simulink model "gm_sampleModel1758_5_sub"  (R2023a)
settings: Solver=VariableStepAuto  StartTime=0.0  StopTime=10.0  RelTol=1e-3
libraries: simulink x1
settings Model: Creator=user1  LastModifiedBy=user1
settings OptimizationCC: BlockReduction=off  ConditionallyExecuteInputs=off
settings DebuggingCC: InheritedTsInSrcMsg=none

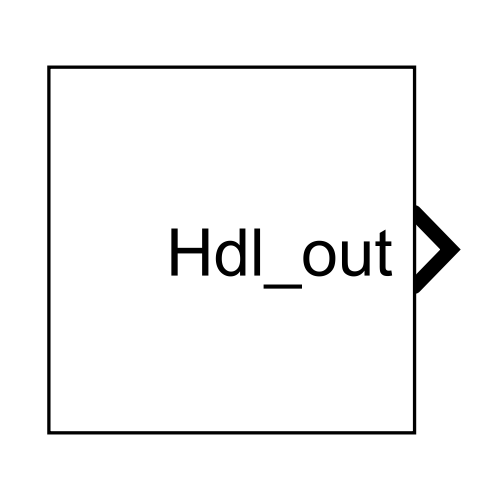
[thumbnail: Simulink's stored preview of the top-level diagram]
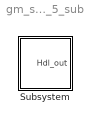
== system gm_sampleModel1758_5_sub ==
  Subsystem : Subsystem

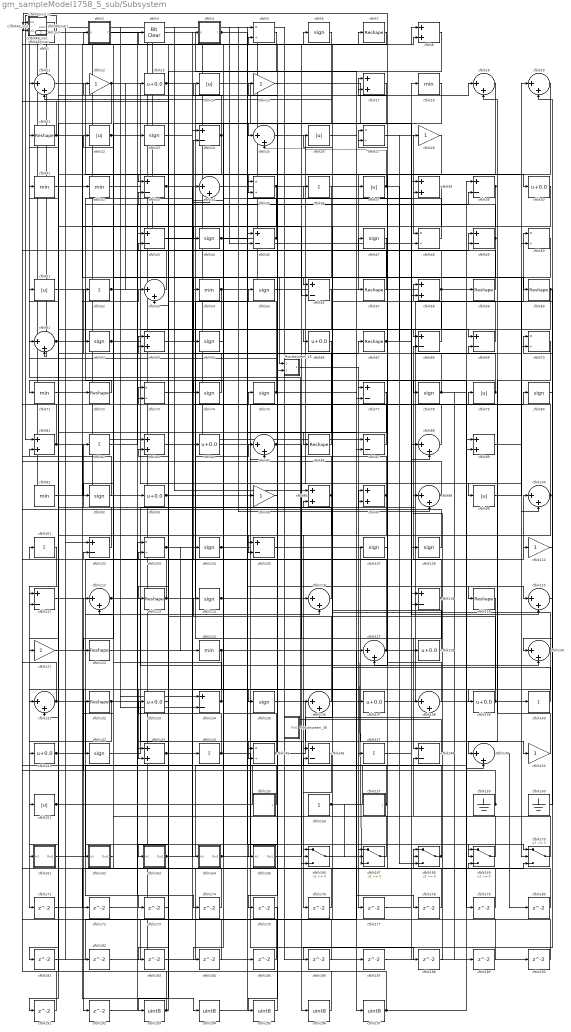
== system gm_sampleModel1758_5_sub/Subsystem ==
  Mysubsystem_38 : Subsystem
  Mysubsystem_45 : Subsystem
  cfblk1 : Logic  AllPortsSameDT=off  OutDataTypeStr=boolean
  cfblk{11,19..20,25,34,53,61,85,88,98,100,112,116,120,127,130..131,136,138,149} (20 alike) : Sum  Inputs=|++  OutDataTypeStr=uint8
  cfblk{36,52,82,101,140,144,147} (7 alike) : Sum  Inputs=+  OutDataTypeStr=uint8
  cfblk{24,33,39,43,45,49,56,68..69,77,87,102,105,111,118,134,146,148} (18 alike) : Sum  Inputs=+-  OutDataTypeStr=uint8
  cfblk{5,27,35,48,50,70,73,103,145} (9 alike) : Product  Inputs=*/  OutDataTypeStr=uint8  RndMeth=Zero  SaturateOnIntegerOverflow=on
  cfblk{6,23,44,47,55,62,64,74..75,78,80,92,104,107..108,114,135,142} (18 alike) : Signum
  cfblk106_inst : Subsystem
  cfblk109_inst : Subsystem
  cfblk10_inst : Subsystem
  cfblk{12,15,28,95,110,121,150} (7 alike) : Gain  OutDataTypeStr=uint8
  cfblk{7,21,57,59..60,67,72,86,113,119,122,132} (12 alike) : Reshape
  cfblk115_inst : Subsystem
  cfblk117_inst : Subsystem
  cfblk{18,31..32,54,71,91,124} (7 alike) : MinMax  OutDataTypeStr=uint8
  cfblk125_inst : Subsystem
  cfblk{13,40,66,84,93,128,133,137,139,141} (10 alike) : Bias  Bias=0.0  SaturateOnIntegerOverflow=off
  cfblk129_inst : Subsystem
  cfblk{14,22,26,37,51,79,99,151} (8 alike) : Abs  OutDataTypeStr=uint8  SaturateOnIntegerOverflow=off
  cfblk{8,17,38,58,63,81,83,89,96..97,143} (11 alike) : Sum  OutDataTypeStr=uint8
  cfblk155 : Subsystem  mask(Counter Limited){uplimit=double(7), tsamp=double(-1)}
      mask prompts: uplimit "Simulink:masks:UpperLimit_MP"; tsamp "Simulink:masks:SampleTime_MP"
      mask help: Simulink:masks:CounterLimited_MD
      mask init:
      | nbits = double(8);
      | tsamp = double(-1);
      | uplimit = double(7);
  cfblk156 : Constant  OutDataTypeStr=uint8  SampleTime=-1
  cfblk157 : Subsystem  mask(Counter Free-Running){NumBits=double(16), tsamp=double(-1)}
      mask prompts: NumBits "Simulink:masks:NumberOfBits_MP"; tsamp "Simulink:masks:SampleTime_MP"
      mask help: Simulink:masks:CounterFreeRunning_MD
  cfblk159 : Ground
  cfblk160 : Ground
  cfblk161 : Subsystem
  cfblk162 : Subsystem
  cfblk163 : Subsystem
  cfblk164 : Subsystem
  cfblk165 : Subsystem
  cfblk{166..170} (5 alike) : Switch  OutDataTypeStr=uint8  SaturateOnIntegerOverflow=off  InputSameDT=off
  cfblk16_inst : Subsystem
  cfblk{171..192} (22 alike) : Delay  SampleTime=1
  cfblk{193..197} (5 alike) : DataTypeConversion  OutDataTypeStr=uint8  SaturateOnIntegerOverflow=off  RndMeth=Floor
  cfblk2 : Subsystem  mask(Detect Fall Nonpositive){vinit=double(0), InputProcessing=Elements as channels (sample based), OutDataTypeStr=uint8}
      mask prompts: vinit "Simulink:masks:InitialCondition_MP"; InputProcessing "Simulink:masks:InputProcessing_MP"; OutDataTypeStr "Simulink:masks:OutputDataType_MP"
      mask help: Simulink:masks:DetectFallNonpositive_MD
      mask init:
      | InputProcessing = 'Elements as channels (sample based)';
      | OutDataTypeStr = 'uint8';
      | vinit = double(0);
      mask TypeOptions InputProcessing: Simulink:masks:ColumnsAsChannelsFrameBased | Simulink:masks:ElementsAsChannelsSampleBased
      mask TypeOptions OutDataTypeStr: Simulink:masks:uint8 | Simulink:masks:boolean
      mask Display: fprintf('U <= 0\n&  NOT\nU/z <= 0')
  cfblk29_inst : Subsystem
  cfblk3 : simulink/Logic and Bit Operations/Bit Clear  iBit=0
      settings: LibrarySourceBlock=|
      | hdlsllib/Logic and Bit
      | Operations/Bit Clear
  cfblk30_inst : Subsystem
  cfblk4 : Subsystem  mask(Detect Rise Nonnegative){vinit=double(0), InputProcessing=Elements as channels (sample based), OutDataTypeStr=uint8}
      mask prompts: vinit "Simulink:masks:InitialCondition_MP"; InputProcessing "Simulink:masks:InputProcessing_MP"; OutDataTypeStr "Simulink:masks:OutputDataType_MP"
      mask help: Simulink:masks:DetectRiseNonnegative_MD
      mask init:
      | InputProcessing = 'Elements as channels (sample based)';
      | OutDataTypeStr = 'uint8';
      | vinit = double(0);
      mask TypeOptions InputProcessing: Simulink:masks:ColumnsAsChannelsFrameBased | Simulink:masks:ElementsAsChannelsSampleBased
      mask TypeOptions OutDataTypeStr: Simulink:masks:uint8 | Simulink:masks:boolean
      mask Display: fprintf('U >= 0\n&  NOT\nU/z >= 0')
  cfblk41_inst : Subsystem
  cfblk42_inst : Subsystem
  cfblk46_inst : Subsystem
  cfblk90_inst : Subsystem
  cfblk94_inst : Subsystem
  cfblk9_inst : Subsystem
  Hdl_out : Outport  OutDataTypeStr=uint8  SampleTime=1
  wires:
  Mysubsystem_38/1(Out1) -> cfblk1/2
  Mysubsystem_45/1(Out1) -> cfblk177/1
  cfblk1/1 -> cfblk81/1
  cfblk10_inst/1(out1) -> cfblk134/1
  cfblk100/1 -> cfblk46_inst/2(in2), cfblk176/1
  cfblk101/1 -> cfblk171/1
  cfblk102/1 -> cfblk82/1
  cfblk103/1 -> cfblk97/1, cfblk55/1, cfblk124/1
  cfblk104/1 -> cfblk85/2, cfblk80/1
  cfblk105/1 -> cfblk150/1
  cfblk106_inst/1(out1) -> cfblk93/1, cfblk102/1
  cfblk107/1 -> cfblk27/1
  cfblk108/1 -> cfblk129_inst/1(in1)
  cfblk109_inst/1(out1) -> cfblk61/2, cfblk117_inst/1(in1), cfblk91/1
  cfblk11/1 -> cfblk40/1
  cfblk110/1 -> cfblk58/1
  cfblk111/1 -> cfblk100/1
  cfblk112/1 -> cfblk130/2, cfblk50/1
  cfblk113/1 -> cfblk85/1, cfblk117_inst/2(in2)
  cfblk114/1 -> cfblk116/1, cfblk110/1
  cfblk115_inst/1(out1) -> cfblk42_inst/2(in2), cfblk185/1
  cfblk116/1 -> cfblk31/1
  cfblk117_inst/1(out1) -> cfblk140/1, cfblk32/1
  cfblk118/1 -> cfblk68/2, cfblk148/1
  cfblk119/1 -> cfblk139/1
  cfblk12/1 -> cfblk149/2, cfblk121/1
  cfblk120/1 -> cfblk186/1
  cfblk121/1 -> cfblk116/2
  cfblk122/1 -> cfblk144/1
  cfblk124/1 -> cfblk167/3, cfblk143/2, cfblk192/1
  cfblk125_inst/1(out1) -> cfblk72/1, cfblk59/1
  cfblk127/1 -> cfblk69/2, cfblk22/1, cfblk73/1
  cfblk128/1 -> cfblk46_inst/1(in1)
  cfblk129_inst/1(out1) -> cfblk87/1, cfblk23/1
  cfblk13/1 -> cfblk25/1, cfblk35/2, cfblk187/1
  cfblk130/1 -> cfblk11/2, cfblk172/1
  cfblk131/1 -> cfblk42_inst/1(in1), cfblk173/1
  cfblk132/1 -> cfblk196/1, cfblk151/1, cfblk181/1
  cfblk133/1 -> cfblk163/1(In1)
  cfblk134/1 -> cfblk83/2, cfblk2/1(U)
  cfblk135/1 -> cfblk147/1
  cfblk136/1 -> cfblk63/1
  cfblk137/1 -> cfblk20/1
  cfblk138/1 -> cfblk115_inst/1(in1)
  cfblk139/1 -> cfblk131/1, cfblk114/1
  cfblk14/1 -> cfblk88/2
  cfblk140/1 -> cfblk6/1
  cfblk141/1 -> cfblk45/2, cfblk24/2, cfblk166/2
  cfblk142/1 -> cfblk79/1
  cfblk143/1 -> cfblk75/1, cfblk67/1
  cfblk144/1 -> cfblk133/1, cfblk188/1
  cfblk145/1 -> cfblk138/2, cfblk104/1
  cfblk146/1 -> cfblk166/1
  cfblk147/1 -> cfblk118/2
  cfblk148/1 -> cfblk101/1
  cfblk149/1 -> cfblk180/1
  cfblk15/1 -> cfblk118/1
  cfblk150/1 -> cfblk19/2
  cfblk151/1 -> cfblk146/2, cfblk18/1
  cfblk155/1(y) -> cfblk112/1
  cfblk156/1 -> cfblk39/1, cfblk167/2
  cfblk157/1(y) -> cfblk24/1, cfblk103/2
  cfblk159/1 -> cfblk30_inst/2(in2), cfblk29_inst/2(in2), cfblk142/1
  cfblk16_inst/1(out1) -> cfblk98/2, cfblk190/1
  cfblk160/1 -> cfblk70/1
  cfblk161/1(Out1) -> cfblk84/1
  cfblk162/1(Out1) -> cfblk132/1
  cfblk163/1(Out1) -> cfblk43/2, cfblk138/1
  cfblk164/1(Out1) -> cfblk97/2, cfblk170/3, cfblk14/1
  cfblk165/1(Out1) -> cfblk7/1
  cfblk166/1 -> cfblk178/1
  cfblk167/1 -> cfblk12/1
  cfblk168/1 -> cfblk16_inst/1(in1), cfblk27/2
  cfblk169/1 -> cfblk34/1
  cfblk17/1 -> cfblk145/2
  cfblk170/1 -> cfblk148/2
  cfblk171/1 -> cfblk168/1
  cfblk172/1 -> cfblk168/2
  cfblk173/1 -> cfblk53/2
  cfblk174/1 -> cfblk102/2
  cfblk175/1 -> cfblk195/1
  cfblk176/1 -> cfblk81/2
  cfblk177/1 -> cfblk88/1
  cfblk178/1 -> cfblk17/1
  cfblk179/1 -> cfblk145/1
  cfblk18/1 -> cfblk112/2
  cfblk180/1 -> cfblk106_inst/1(in1)
  cfblk181/1 -> cfblk34/2
  cfblk182/1 -> cfblk127/1
  cfblk183/1 -> cfblk169/3
  cfblk184/1 -> cfblk16_inst/2(in2)
  cfblk185/1 -> cfblk45/1
  cfblk186/1 -> cfblk41_inst/2(in2)
  cfblk187/1 -> cfblk49/1
  cfblk188/1 -> cfblk98/1
  cfblk189/1 -> cfblk94_inst/2(in2)
  cfblk19/1 -> cfblk57/1
  cfblk190/1 -> cfblk96/2
  cfblk191/1 -> cfblk1/1
  cfblk192/1 -> cfblk103/1
  cfblk193/1 -> cfblk94_inst/1(in1), cfblk73/2
  cfblk194/1 -> cfblk5/1
  cfblk195/1 -> cfblk5/2
  cfblk196/1 -> cfblk3/1
  cfblk197/1 -> cfblk89/2, cfblk51/1
  cfblk2/1(Y) -> cfblk174/1
  cfblk20/1 -> cfblk127/2
  cfblk21/1 -> cfblk44/1, cfblk109_inst/2(in2)
  cfblk22/1 -> cfblk58/2, cfblk169/2, cfblk169/1
  cfblk23/1 -> cfblk17/2
  cfblk24/1 -> cfblk33/1, cfblk115_inst/2(in2)
  cfblk25/1 -> cfblk100/2
  cfblk26/1 -> cfblk170/1
  cfblk27/1 -> cfblk48/1
  cfblk28/1 -> cfblk141/1
  cfblk29_inst/1(out1) -> cfblk37/1
  cfblk3/1 -> cfblk197/1
  cfblk30_inst/1(out1) -> cfblk182/1
  cfblk31/1 -> cfblk56/1
  cfblk32/1 -> cfblk56/2
  cfblk33/1 -> cfblk38/2, cfblk167/1
  cfblk34/1 -> cfblk119/1
  cfblk35/1 -> cfblk170/2, cfblk131/2, cfblk122/1, cfblk108/1
  cfblk36/1 -> cfblk92/1
  cfblk37/1 -> cfblk25/2, cfblk168/3
  cfblk38/1 -> cfblk135/1
  cfblk39/1 -> cfblk136/2, cfblk105/2
  cfblk4/1(Y) -> cfblk86/1, cfblk78/1, cfblk68/1, cfblk166/3
  cfblk40/1 -> cfblk66/1
  cfblk41_inst/1(out1) -> cfblk96/1
  cfblk42_inst/1(out1) -> cfblk83/1, cfblk134/2
  cfblk43/1 -> cfblk136/1
  cfblk44/1 -> cfblk87/2, cfblk69/1
  cfblk45/1 -> cfblk129_inst/2(in2), Hdl_out/1
  cfblk46_inst/1(out1) -> cfblk9_inst/1(in1), cfblk10_inst/1(in1)
  cfblk47/1 -> cfblk64/1
  cfblk48/1 -> cfblk30_inst/1(in1)
  cfblk49/1 -> cfblk74/1, cfblk33/2
  cfblk5/1 -> cfblk193/1
  cfblk50/1 -> Mysubsystem_45/1(In1)
  cfblk51/1 -> cfblk179/1
  cfblk52/1 -> cfblk77/2, cfblk13/1
  cfblk53/1 -> cfblk109_inst/1(in1)
  cfblk54/1 -> cfblk60/1, cfblk111/2
  cfblk55/1 -> cfblk8/2
  cfblk56/1 -> cfblk111/1
  cfblk57/1 -> cfblk21/1
  cfblk58/1 -> cfblk9_inst/2(in2), cfblk107/1, cfblk183/1
  cfblk59/1 -> cfblk15/1
  cfblk6/1 -> cfblk54/1
  cfblk60/1 -> cfblk143/1, cfblk130/1
  cfblk61/1 -> cfblk35/1, cfblk4/1(U)
  cfblk62/1 -> cfblk39/2, cfblk164/1(In1)
  cfblk63/1 -> cfblk146/1
  cfblk64/1 -> cfblk184/1
  cfblk66/1 -> cfblk161/1(In1)
  cfblk67/1 -> cfblk120/2, cfblk28/1
  cfblk68/1 -> cfblk26/1
  cfblk69/1 -> cfblk47/1
  cfblk7/1 -> cfblk90_inst/2(in2)
  cfblk70/1 -> cfblk149/1
  cfblk71/1 -> cfblk53/1
  cfblk72/1 -> cfblk71/1
  cfblk73/1 -> cfblk99/1
  cfblk74/1 -> cfblk29_inst/1(in1)
  cfblk75/1 -> cfblk120/1, cfblk11/1
  cfblk77/1 -> cfblk165/1(In1)
  cfblk78/1 -> cfblk89/1, cfblk43/1, cfblk189/1
  cfblk79/1 -> cfblk77/1, cfblk63/2
  cfblk8/1 -> cfblk113/1
  cfblk80/1 -> cfblk20/2
  cfblk81/1 -> cfblk194/1, cfblk125_inst/2(in2)
  cfblk82/1 -> cfblk49/2
  cfblk83/1 -> cfblk95/1
  cfblk84/1 -> cfblk38/1
  cfblk85/1 -> cfblk128/1, Mysubsystem_45/2(In2)
  cfblk86/1 -> cfblk52/1
  cfblk87/1 -> cfblk90_inst/1(in1)
  cfblk88/1 -> cfblk41_inst/1(in1)
  cfblk89/1 -> cfblk70/2
  cfblk9_inst/1(out1) -> cfblk162/1(In1)
  cfblk90_inst/1(out1) -> cfblk48/2
  cfblk91/1 -> cfblk8/1
  cfblk92/1 -> cfblk10_inst/2(in2)
  cfblk93/1 -> cfblk19/1, cfblk137/1
  cfblk94_inst/1(out1) -> cfblk62/1
  cfblk95/1 -> cfblk175/1
  cfblk96/1 -> cfblk106_inst/2(in2), cfblk105/1
  cfblk97/1 -> cfblk61/1, cfblk191/1
  cfblk98/1 -> cfblk125_inst/1(in1), cfblk36/1
  cfblk99/1 -> cfblk50/2

== system gm_sampleModel1758_5_sub/Subsystem/Mysubsystem_38 ==
  cfblk123 : Abs  SaturateOnIntegerOverflow=off
  cfblk158 : Ground
  Out1 : Outport  SampleTime=1
  wires:
  cfblk123/1 -> Out1/1
  cfblk158/1 -> cfblk123/1

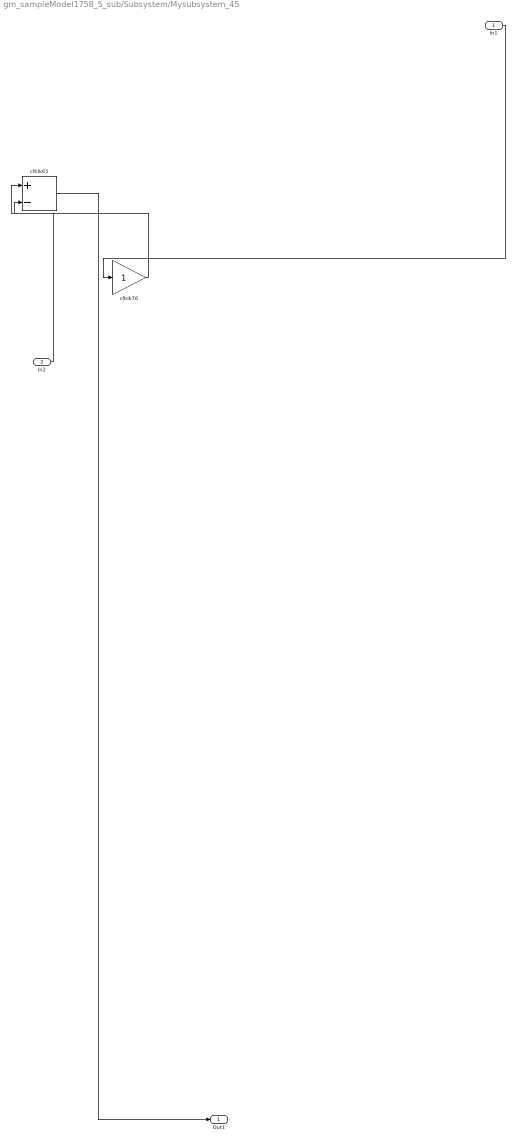
== system gm_sampleModel1758_5_sub/Subsystem/Mysubsystem_45 ==
  In1 : Inport  OutDataTypeStr=uint8  PortDimensions=1  SampleTime=1
  In2 : Inport  Port=2  OutDataTypeStr=uint8  PortDimensions=1  SampleTime=1
  cfblk65 : Sum  Inputs=+-
  cfblk76 : Gain
  Out1 : Outport  SampleTime=1
  wires:
  In1/1 -> cfblk76/1
  In2/1 -> cfblk65/2
  cfblk65/1 -> Out1/1
  cfblk76/1 -> cfblk65/1

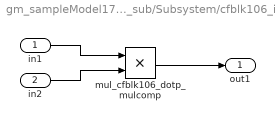
== system gm_sampleModel1758_5_sub/Subsystem/cfblk106_inst ==
  in1 : Inport  OutDataTypeStr=uint8  SampleTime=1
  in2 : Inport  Port=2  OutDataTypeStr=uint8  SampleTime=1
  mul_cfblk106_dotp_mulcomp : Product  Inputs=**  OutDataTypeStr=uint8  SampleTime=1
  out1 : Outport  OutDataTypeStr=uint8  SampleTime=1
  wires:
  in1/1 -> mul_cfblk106_dotp_mulcomp/1
  in2/1 -> mul_cfblk106_dotp_mulcomp/2
  mul_cfblk106_dotp_mulcomp/1 -> out1/1

== system gm_sampleModel1758_5_sub/Subsystem/cfblk109_inst ==
  in1 : Inport  OutDataTypeStr=uint8  SampleTime=1
  in2 : Inport  Port=2  OutDataTypeStr=uint8  SampleTime=1
  mul_cfblk109_dotp_mulcomp : Product  Inputs=**  OutDataTypeStr=uint8  SampleTime=1
  out1 : Outport  OutDataTypeStr=uint8  SampleTime=1
  wires:
  in1/1 -> mul_cfblk109_dotp_mulcomp/1
  in2/1 -> mul_cfblk109_dotp_mulcomp/2
  mul_cfblk109_dotp_mulcomp/1 -> out1/1

== system gm_sampleModel1758_5_sub/Subsystem/cfblk10_inst ==
  in1 : Inport  OutDataTypeStr=uint8  SampleTime=1
  in2 : Inport  Port=2  OutDataTypeStr=uint8  SampleTime=1
  mul_cfblk10_dotp_mulcomp : Product  Inputs=**  OutDataTypeStr=uint8  SampleTime=1
  out1 : Outport  OutDataTypeStr=uint8  SampleTime=1
  wires:
  in1/1 -> mul_cfblk10_dotp_mulcomp/1
  in2/1 -> mul_cfblk10_dotp_mulcomp/2
  mul_cfblk10_dotp_mulcomp/1 -> out1/1

== system gm_sampleModel1758_5_sub/Subsystem/cfblk115_inst ==
  in1 : Inport  OutDataTypeStr=uint8  SampleTime=1
  in2 : Inport  Port=2  OutDataTypeStr=uint8  SampleTime=1
  mul_cfblk115_dotp_mulcomp : Product  Inputs=**  OutDataTypeStr=uint8  SampleTime=1
  out1 : Outport  OutDataTypeStr=uint8  SampleTime=1
  wires:
  in1/1 -> mul_cfblk115_dotp_mulcomp/1
  in2/1 -> mul_cfblk115_dotp_mulcomp/2
  mul_cfblk115_dotp_mulcomp/1 -> out1/1

== system gm_sampleModel1758_5_sub/Subsystem/cfblk117_inst ==
  in1 : Inport  OutDataTypeStr=uint8  SampleTime=1
  in2 : Inport  Port=2  OutDataTypeStr=uint8  SampleTime=1
  mul_cfblk117_dotp_mulcomp : Product  Inputs=**  OutDataTypeStr=uint8  SampleTime=1
  out1 : Outport  OutDataTypeStr=uint8  SampleTime=1
  wires:
  in1/1 -> mul_cfblk117_dotp_mulcomp/1
  in2/1 -> mul_cfblk117_dotp_mulcomp/2
  mul_cfblk117_dotp_mulcomp/1 -> out1/1

== system gm_sampleModel1758_5_sub/Subsystem/cfblk125_inst ==
  in1 : Inport  OutDataTypeStr=uint8  SampleTime=1
  in2 : Inport  Port=2  OutDataTypeStr=uint8  SampleTime=1
  mul_cfblk125_dotp_mulcomp : Product  Inputs=**  OutDataTypeStr=uint8  SampleTime=1
  out1 : Outport  OutDataTypeStr=uint8  SampleTime=1
  wires:
  in1/1 -> mul_cfblk125_dotp_mulcomp/1
  in2/1 -> mul_cfblk125_dotp_mulcomp/2
  mul_cfblk125_dotp_mulcomp/1 -> out1/1

== system gm_sampleModel1758_5_sub/Subsystem/cfblk129_inst ==
  in1 : Inport  OutDataTypeStr=uint8  SampleTime=1
  in2 : Inport  Port=2  OutDataTypeStr=uint8  SampleTime=1
  mul_cfblk129_dotp_mulcomp : Product  Inputs=**  OutDataTypeStr=uint8  SampleTime=1
  out1 : Outport  OutDataTypeStr=uint8  SampleTime=1
  wires:
  in1/1 -> mul_cfblk129_dotp_mulcomp/1
  in2/1 -> mul_cfblk129_dotp_mulcomp/2
  mul_cfblk129_dotp_mulcomp/1 -> out1/1

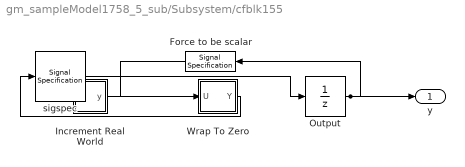
== system gm_sampleModel1758_5_sub/Subsystem/cfblk155 ==
  Force to be scalar : SignalSpecification  DisableCoverage=on  Dimensions=1
  Increment Real World : Subsystem  mask(Real World Value Increment){}
      mask help: Simulink:masks:RealWorldValueIncrement_MD
      mask Display: disp('V++')
  Output : UnitDelay  InitialCondition=0.0  SampleTime=tsamp  HasFrameUpgradeWarning=on
  Wrap To Zero : Subsystem  mask(Wrap To Zero){Threshold=double(7)}
      mask prompts: Threshold "Simulink:masks:Threshold_MP"
      mask help: Simulink:masks:WrapToZero_MD
  sigspec : SignalSpecification  OutDataTypeStr=uint8  Dimensions=1
  y : Outport  SampleTime=1
  wires:
  Force to be scalar/1 -> Increment Real World/1(u)
  Increment Real World/1(y) -> Wrap To Zero/1(U)
  Output/1 -> Force to be scalar/1, y/1
  Wrap To Zero/1(Y) -> sigspec/1
  sigspec/1 -> Output/1

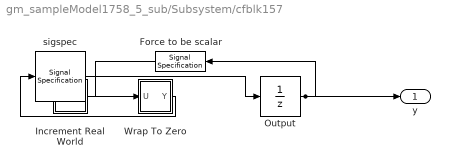
== system gm_sampleModel1758_5_sub/Subsystem/cfblk157 ==
  Force to be scalar : SignalSpecification  DisableCoverage=on  Dimensions=1
  Increment Real World : Subsystem  mask(Real World Value Increment){}
      mask help: Simulink:masks:RealWorldValueIncrement_MD
      mask Display: disp('V++')
  Output : UnitDelay  InitialCondition=0.0  SampleTime=tsamp  HasFrameUpgradeWarning=on
  Wrap To Zero : Subsystem  mask(Wrap To Zero){Threshold=double(65535)}
      mask prompts: Threshold "Simulink:masks:Threshold_MP"
      mask help: Simulink:masks:WrapToZero_MD
  sigspec : SignalSpecification  OutDataTypeStr=uint16  Dimensions=1
  y : Outport  SampleTime=1
  wires:
  Force to be scalar/1 -> Increment Real World/1(u)
  Increment Real World/1(y) -> Wrap To Zero/1(U)
  Output/1 -> Force to be scalar/1, y/1
  Wrap To Zero/1(Y) -> sigspec/1
  sigspec/1 -> Output/1

== system gm_sampleModel1758_5_sub/Subsystem/cfblk161 ==
  In1 : Inport  OutDataTypeStr=uint8  PortDimensions=1  SampleTime=1
  Out1 : Outport  SampleTime=1
  wires:
  In1/1 -> Out1/1

== system gm_sampleModel1758_5_sub/Subsystem/cfblk162 ==
  In1 : Inport  OutDataTypeStr=uint8  PortDimensions=1  SampleTime=1
  Out1 : Outport  SampleTime=1
  wires:
  In1/1 -> Out1/1

== system gm_sampleModel1758_5_sub/Subsystem/cfblk163 ==
  In1 : Inport  OutDataTypeStr=uint8  PortDimensions=1  SampleTime=1
  Out1 : Outport  SampleTime=1
  wires:
  In1/1 -> Out1/1

== system gm_sampleModel1758_5_sub/Subsystem/cfblk164 ==
  In1 : Inport  OutDataTypeStr=uint8  PortDimensions=1  SampleTime=1
  Out1 : Outport  SampleTime=1
  wires:
  In1/1 -> Out1/1

== system gm_sampleModel1758_5_sub/Subsystem/cfblk165 ==
  In1 : Inport  OutDataTypeStr=uint8  PortDimensions=1  SampleTime=1
  Out1 : Outport  SampleTime=1
  wires:
  In1/1 -> Out1/1

== system gm_sampleModel1758_5_sub/Subsystem/cfblk16_inst ==
  in1 : Inport  OutDataTypeStr=uint8  SampleTime=1
  in2 : Inport  Port=2  OutDataTypeStr=uint8  SampleTime=1
  mul_cfblk16_dotp_mulcomp : Product  Inputs=**  OutDataTypeStr=uint8  SampleTime=1
  out1 : Outport  OutDataTypeStr=uint8  SampleTime=1
  wires:
  in1/1 -> mul_cfblk16_dotp_mulcomp/1
  in2/1 -> mul_cfblk16_dotp_mulcomp/2
  mul_cfblk16_dotp_mulcomp/1 -> out1/1

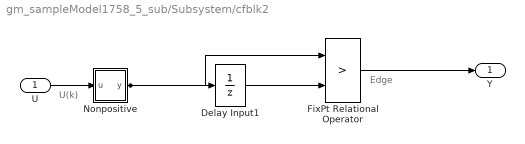
== system gm_sampleModel1758_5_sub/Subsystem/cfblk2 ==
  note: U(k)
  note: Edge
  U : Inport  OutDataTypeStr=uint8  SampleTime=1
  Delay Input1 : UnitDelay  Description=Store in Global RAM  DisableCoverage=on  InitialCondition=vinit  SampleTime=-1  HasFrameUpgradeWarning=on
  FixPt Relational Operator : RelationalOperator  Operator=>  OutDataTypeStr=fixdt(0, 8)  ZeroCross=off  InputSameDT=off
  Nonpositive : Subsystem  mask(Compare To Zero){relop=<=, OutDataTypeStr=boolean, ZeroCross=off}
      mask prompts: relop "Simulink:masks:Operator_MP"; OutDataTypeStr "Simulink:masks:OutputDataType_MP"; ZeroCross "Simulink:masks:EnableZerocrossingDetection_MP"
      mask help: Simulink:masks:CompareToZero_MD
      mask init:
      | OutDataTypeStr = 'boolean';
      | ZeroCross = 'off';
      | blkName = 'sampleModel1758_5_sub/Subsystem/cfblk2/Nonpositive';
      | relop = '<=';
      | setValue = 'boolean';
      mask TypeOptions relop: == | ~= | < | <= | >= | >
      mask TypeOptions OutDataTypeStr: Simulink:masks:uint8 | Simulink:masks:boolean
      mask Callback ZeroCross: sl('zeroCrossEnable', gcbh);
      mask Display: disp([relop,' 0'])
  Y : Outport  SampleTime=1
  wires:
  U/1 -> Nonpositive/1(u)
  Delay Input1/1 -> FixPt Relational Operator/2
  FixPt Relational Operator/1 -> Y/1
  Nonpositive/1(y) -> FixPt Relational Operator/1, Delay Input1/1

== system gm_sampleModel1758_5_sub/Subsystem/cfblk29_inst ==
  in1 : Inport  OutDataTypeStr=uint8  SampleTime=1
  in2 : Inport  Port=2  OutDataTypeStr=uint8  SampleTime=1
  mul_cfblk29_dotp_mulcomp : Product  Inputs=**  OutDataTypeStr=uint8  SampleTime=1
  out1 : Outport  OutDataTypeStr=uint8  SampleTime=1
  wires:
  in1/1 -> mul_cfblk29_dotp_mulcomp/1
  in2/1 -> mul_cfblk29_dotp_mulcomp/2
  mul_cfblk29_dotp_mulcomp/1 -> out1/1

== system gm_sampleModel1758_5_sub/Subsystem/cfblk30_inst ==
  in1 : Inport  OutDataTypeStr=uint8  SampleTime=1
  in2 : Inport  Port=2  OutDataTypeStr=uint8  SampleTime=1
  mul_cfblk30_dotp_mulcomp : Product  Inputs=**  OutDataTypeStr=uint8  SampleTime=1
  out1 : Outport  OutDataTypeStr=uint8  SampleTime=1
  wires:
  in1/1 -> mul_cfblk30_dotp_mulcomp/1
  in2/1 -> mul_cfblk30_dotp_mulcomp/2
  mul_cfblk30_dotp_mulcomp/1 -> out1/1

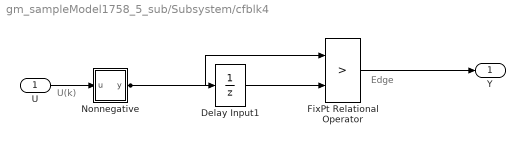
== system gm_sampleModel1758_5_sub/Subsystem/cfblk4 ==
  note: U(k)
  note: Edge
  U : Inport  OutDataTypeStr=uint8  SampleTime=1
  Delay Input1 : UnitDelay  Description=Store in Global RAM  DisableCoverage=on  InitialCondition=vinit  SampleTime=-1  HasFrameUpgradeWarning=on
  FixPt Relational Operator : RelationalOperator  Operator=>  OutDataTypeStr=fixdt(0, 8)  ZeroCross=off  InputSameDT=off
  Nonnegative : Subsystem  mask(Compare To Zero){relop=>=, OutDataTypeStr=boolean, ZeroCross=off}
      mask prompts: relop "Simulink:masks:Operator_MP"; OutDataTypeStr "Simulink:masks:OutputDataType_MP"; ZeroCross "Simulink:masks:EnableZerocrossingDetection_MP"
      mask help: Simulink:masks:CompareToZero_MD
      mask init:
      | OutDataTypeStr = 'boolean';
      | ZeroCross = 'off';
      | blkName = 'sampleModel1758_5_sub/Subsystem/cfblk4/Nonnegative';
      | relop = '>=';
      | setValue = 'boolean';
      mask TypeOptions relop: == | ~= | < | <= | >= | >
      mask TypeOptions OutDataTypeStr: Simulink:masks:uint8 | Simulink:masks:boolean
      mask Callback ZeroCross: sl('zeroCrossEnable', gcbh);
      mask Display: disp([relop,' 0'])
  Y : Outport  SampleTime=1
  wires:
  U/1 -> Nonnegative/1(u)
  Delay Input1/1 -> FixPt Relational Operator/2
  FixPt Relational Operator/1 -> Y/1
  Nonnegative/1(y) -> FixPt Relational Operator/1, Delay Input1/1

== system gm_sampleModel1758_5_sub/Subsystem/cfblk41_inst ==
  in1 : Inport  OutDataTypeStr=uint8  SampleTime=1
  in2 : Inport  Port=2  OutDataTypeStr=uint8  SampleTime=1
  mul_cfblk41_dotp_mulcomp : Product  Inputs=**  OutDataTypeStr=uint8  SampleTime=1
  out1 : Outport  OutDataTypeStr=uint8  SampleTime=1
  wires:
  in1/1 -> mul_cfblk41_dotp_mulcomp/1
  in2/1 -> mul_cfblk41_dotp_mulcomp/2
  mul_cfblk41_dotp_mulcomp/1 -> out1/1

== system gm_sampleModel1758_5_sub/Subsystem/cfblk42_inst ==
  in1 : Inport  OutDataTypeStr=uint8  SampleTime=1
  in2 : Inport  Port=2  OutDataTypeStr=uint8  SampleTime=1
  mul_cfblk42_dotp_mulcomp : Product  Inputs=**  OutDataTypeStr=uint8  SampleTime=1
  out1 : Outport  OutDataTypeStr=uint8  SampleTime=1
  wires:
  in1/1 -> mul_cfblk42_dotp_mulcomp/1
  in2/1 -> mul_cfblk42_dotp_mulcomp/2
  mul_cfblk42_dotp_mulcomp/1 -> out1/1

== system gm_sampleModel1758_5_sub/Subsystem/cfblk46_inst ==
  in1 : Inport  OutDataTypeStr=uint8  SampleTime=1
  in2 : Inport  Port=2  OutDataTypeStr=uint8  SampleTime=1
  mul_cfblk46_dotp_mulcomp : Product  Inputs=**  OutDataTypeStr=uint8  SampleTime=1
  out1 : Outport  OutDataTypeStr=uint8  SampleTime=1
  wires:
  in1/1 -> mul_cfblk46_dotp_mulcomp/1
  in2/1 -> mul_cfblk46_dotp_mulcomp/2
  mul_cfblk46_dotp_mulcomp/1 -> out1/1

== system gm_sampleModel1758_5_sub/Subsystem/cfblk90_inst ==
  in1 : Inport  OutDataTypeStr=uint8  SampleTime=1
  in2 : Inport  Port=2  OutDataTypeStr=uint8  SampleTime=1
  mul_cfblk90_dotp_mulcomp : Product  Inputs=**  OutDataTypeStr=uint8  SampleTime=1
  out1 : Outport  OutDataTypeStr=uint8  SampleTime=1
  wires:
  in1/1 -> mul_cfblk90_dotp_mulcomp/1
  in2/1 -> mul_cfblk90_dotp_mulcomp/2
  mul_cfblk90_dotp_mulcomp/1 -> out1/1

== system gm_sampleModel1758_5_sub/Subsystem/cfblk94_inst ==
  in1 : Inport  OutDataTypeStr=uint8  SampleTime=1
  in2 : Inport  Port=2  OutDataTypeStr=uint8  SampleTime=1
  mul_cfblk94_dotp_mulcomp : Product  Inputs=**  OutDataTypeStr=uint8  SampleTime=1
  out1 : Outport  OutDataTypeStr=uint8  SampleTime=1
  wires:
  in1/1 -> mul_cfblk94_dotp_mulcomp/1
  in2/1 -> mul_cfblk94_dotp_mulcomp/2
  mul_cfblk94_dotp_mulcomp/1 -> out1/1

== system gm_sampleModel1758_5_sub/Subsystem/cfblk9_inst ==
  in1 : Inport  OutDataTypeStr=uint8  SampleTime=1
  in2 : Inport  Port=2  OutDataTypeStr=uint8  SampleTime=1
  mul_cfblk9_dotp_mulcomp : Product  Inputs=**  OutDataTypeStr=uint8  SampleTime=1
  out1 : Outport  OutDataTypeStr=uint8  SampleTime=1
  wires:
  in1/1 -> mul_cfblk9_dotp_mulcomp/1
  in2/1 -> mul_cfblk9_dotp_mulcomp/2
  mul_cfblk9_dotp_mulcomp/1 -> out1/1

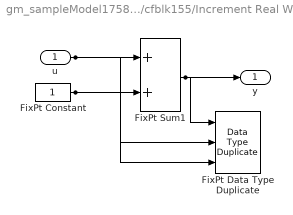
== system gm_sampleModel1758_5_sub/Subsystem/cfblk155/Increment Real World ==
  u : Inport  OutDataTypeStr=uint8  SampleTime=1
  FixPt Constant : Constant  DisableCoverage=on  OutDataTypeStr=Inherit: Inherit via back propagation  SampleTime=-1
  FixPt Data Type Duplicate : DataTypeDuplicate  DisableCoverage=on  NumInputPorts=3
  FixPt Sum1 : Sum  InputSameDT=on  OutDataTypeStr=Inherit: Inherit via back propagation  LockScale=on
  y : Outport  SampleTime=1
  wires:
  u/1 -> FixPt Sum1/1, FixPt Data Type Duplicate/2
  FixPt Constant/1 -> FixPt Sum1/2, FixPt Data Type Duplicate/3
  FixPt Sum1/1 -> FixPt Data Type Duplicate/1, y/1

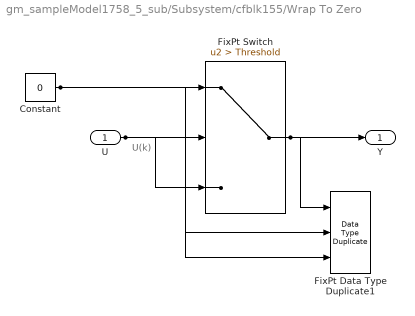
== system gm_sampleModel1758_5_sub/Subsystem/cfblk155/Wrap To Zero ==
  note: U(k)
  U : Inport  OutDataTypeStr=uint8  SampleTime=1
  Constant : Constant  DisableCoverage=on  Value=0  OutDataTypeStr=Inherit: Inherit via back propagation  SampleTime=-1
  FixPt Data Type Duplicate1 : DataTypeDuplicate  DisableCoverage=on  NumInputPorts=3
  FixPt Switch : Switch  Criteria=u2 > Threshold  Threshold=Threshold  OutDataTypeStr=Inherit: Inherit via back propagation  ZeroCross=off  SaturateOnIntegerOverflow=off  InputSameDT=off
  Y : Outport  SampleTime=1
  wires:
  U/1 -> FixPt Switch/3, FixPt Switch/2, FixPt Data Type Duplicate1/2
  Constant/1 -> FixPt Switch/1, FixPt Data Type Duplicate1/3
  FixPt Switch/1 -> FixPt Data Type Duplicate1/1, Y/1

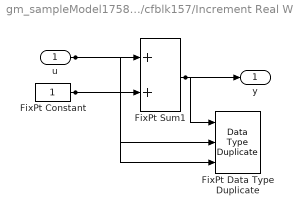
== system gm_sampleModel1758_5_sub/Subsystem/cfblk157/Increment Real World ==
  u : Inport  OutDataTypeStr=uint16  SampleTime=1
  FixPt Constant : Constant  DisableCoverage=on  OutDataTypeStr=Inherit: Inherit via back propagation  SampleTime=-1
  FixPt Data Type Duplicate : DataTypeDuplicate  DisableCoverage=on  NumInputPorts=3
  FixPt Sum1 : Sum  InputSameDT=on  OutDataTypeStr=Inherit: Inherit via back propagation  LockScale=on
  y : Outport  SampleTime=1
  wires:
  u/1 -> FixPt Sum1/1, FixPt Data Type Duplicate/2
  FixPt Constant/1 -> FixPt Sum1/2, FixPt Data Type Duplicate/3
  FixPt Sum1/1 -> FixPt Data Type Duplicate/1, y/1

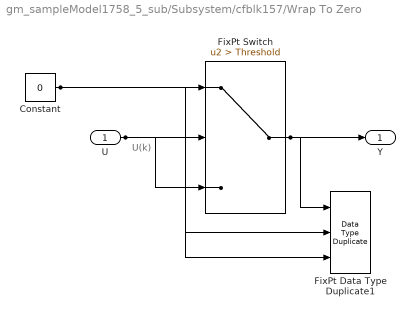
== system gm_sampleModel1758_5_sub/Subsystem/cfblk157/Wrap To Zero ==
  note: U(k)
  U : Inport  OutDataTypeStr=uint16  SampleTime=1
  Constant : Constant  DisableCoverage=on  Value=0  OutDataTypeStr=Inherit: Inherit via back propagation  SampleTime=-1
  FixPt Data Type Duplicate1 : DataTypeDuplicate  DisableCoverage=on  NumInputPorts=3
  FixPt Switch : Switch  Criteria=u2 > Threshold  Threshold=Threshold  OutDataTypeStr=Inherit: Inherit via back propagation  ZeroCross=off  SaturateOnIntegerOverflow=off  InputSameDT=off
  Y : Outport  SampleTime=1
  wires:
  U/1 -> FixPt Switch/3, FixPt Switch/2, FixPt Data Type Duplicate1/2
  Constant/1 -> FixPt Switch/1, FixPt Data Type Duplicate1/3
  FixPt Switch/1 -> FixPt Data Type Duplicate1/1, Y/1

== system gm_sampleModel1758_5_sub/Subsystem/cfblk2/Nonpositive ==
  u : Inport  OutDataTypeStr=uint8  SampleTime=1
  Compare : RelationalOperator  Operator=<=  OutDataTypeStr=boolean  ZeroCross=off
  Constant : Constant  DisableCoverage=on  Value=0  OutDataTypeStr=Inherit: Inherit via back propagation  SampleTime=-1  PreserveConstantTs=on
  y : Outport  SampleTime=1
  wires:
  u/1 -> Compare/1
  Compare/1 -> y/1
  Constant/1 -> Compare/2

== system gm_sampleModel1758_5_sub/Subsystem/cfblk4/Nonnegative ==
  u : Inport  OutDataTypeStr=uint8  SampleTime=1
  Compare : RelationalOperator  OutDataTypeStr=boolean  ZeroCross=off
  Constant : Constant  DisableCoverage=on  Value=0  OutDataTypeStr=Inherit: Inherit via back propagation  SampleTime=-1  PreserveConstantTs=on
  y : Outport  SampleTime=1
  wires:
  u/1 -> Compare/1
  Compare/1 -> y/1
  Constant/1 -> Compare/2
